simulink model "lab5"  (R2016a)
settings: Solver=VariableStepAuto  StartTime=0.0  StopTime=10.0  RelTol=1e-3
settings Model: Creator=sk42595  LastModifiedBy=sk42595

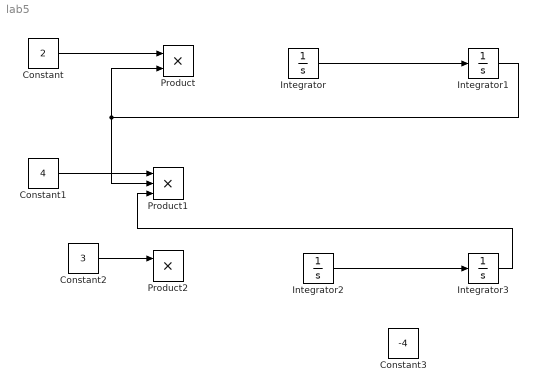
== system lab5 ==
  Constant : Constant  Value=2
  Constant1 : Constant  Value=4
  Constant2 : Constant  Value=3
  Constant3 : Constant  Value=-4
  Integrator{,1..3} (4 alike) : Integrator
  Product : Product
  Product1 : Product  Inputs=3
  Product2 : Product
  wires:
  Integrator/1 -> Integrator1/1
  Integrator2/1 -> Integrator3/1
  Constant/1 -> Product/1
  Integrator1/1 -> Product/2, Product1/2
  Constant1/1 -> Product1/1
  Integrator3/1 -> Product1/3
  Constant2/1 -> Product2/1
